simulink model "SlewAndControlConstrained_Controller_unit_test_2"  (R2018b)
settings: Solver=FixedStepAuto  StartTime=0.0  StopTime=75  FixedStep=simParams.sample_time_s  RelTol=1e-3
undefined symbols (not defined in the file or in its folder): simParams
libraries: sharedutil x1, SlewAndControlConstrained_Controller_lib x1, control_command_generation_lib x1, satelliteDynamics_lib x1
settings Model: Creator=colem  LastModifiedBy=colem

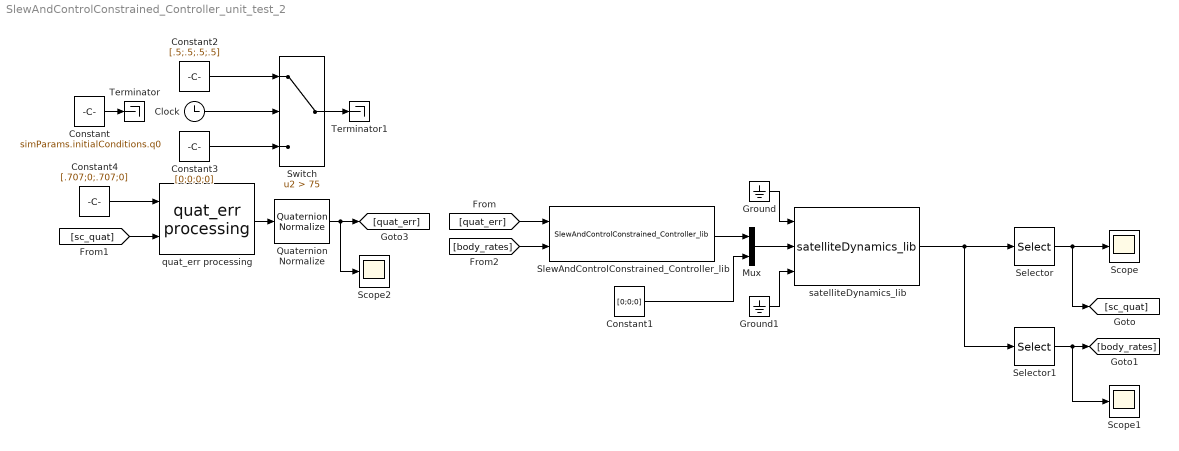
== system SlewAndControlConstrained_Controller_unit_test_2 ==
  Clock : Clock
  Constant : Constant  Value=simParams.initialConditions.q0
  Constant1 : Constant  Value=[0;0;0]
  Constant2 : Constant  Value=[.5;.5;.5;.5]
  Constant3 : Constant  Value=[0;0;0;0]
  Constant4 : Constant  Value=[.707;0;.707;0]
  Ground : Ground
  Ground1 : Ground
  Mux : Mux  Inputs=[3 3]
  Quaternion Normalize : sharedutil/Quaternion Normalize  aMode=aMode
      settings: SourceProductName=Aerospace Blockset  SourceProductBaseCode=AE
  Scope : Scope
  Scope1 : Scope
  Scope2 : Scope
  Selector : Selector  InputPortWidth=13  IndexOptions=Index vector (dialog)  Indices=[7 8 9 10]  OutputSizes=1
  Selector1 : Selector  InputPortWidth=13  IndexOptions=Index vector (dialog)  Indices=[11 12 13]  OutputSizes=1
  SlewAndControlConstrained_Controller_lib : SlewAndControlConstrained_Controller_lib/SlewAndControlConstrained_Controller_lib  SystemSampleTime=-1
  Switch : Switch  Criteria=u2 > Threshold  Threshold=75
  Terminator : Terminator
  Terminator1 : Terminator
  quat_err processing : control_command_generation_lib/control_command_generation_lib/quat_err processing  SystemSampleTime=-1
  satelliteDynamics_lib : satelliteDynamics_lib/satelliteDynamics_lib  SystemSampleTime=-1
  wires:
  Constant/1 -> Terminator/1
  [sc_quat] -> quat_err processing/2
  [quat_err] -> SlewAndControlConstrained_Controller_lib/1
  satelliteDynamics_lib/1 -> Selector1/1, Selector/1
  Selector/1 -> [sc_quat], Scope/1
  Selector1/1 -> Scope1/1, [body_rates]
  [body_rates] -> SlewAndControlConstrained_Controller_lib/2
  Ground/1 -> satelliteDynamics_lib/1
  Ground1/1 -> satelliteDynamics_lib/3
  Constant1/1 -> Mux/2
  SlewAndControlConstrained_Controller_lib/1 -> Mux/1
  Mux/1 -> satelliteDynamics_lib/2
  Constant2/1 -> Switch/1
  Constant3/1 -> Switch/3
  Clock/1 -> Switch/2
  Switch/1 -> Terminator1/1
  Constant4/1 -> quat_err processing/1
  quat_err processing/1 -> Quaternion Normalize/1
  Quaternion Normalize/1 -> Scope2/1, [quat_err]
